simulink model "stm32f0_can_slave_demo"  (Simulink 7.3)
settings: Solver=ode3  SolverMode=SingleTasking  StartTime=0.0  StopTime=10.0  RelTol=1e-3
PreLoadFcn:
  | waijung.modelPreload; % Required for working with Waijung Blockset. Do not remove.
undefined symbols (not defined in the file): current, LQFP48, STM32F072CB, voltage
libraries: stm32f0_can_lib x3, simulink x2, stm32f0_adc_lib x1, stm32f0_device_config_lib x1
CloseFcn:
  | waijung.modelClose; % Required for working with Waijung Blockset. Do not remove.
settings Model: Creator=Krisada  LastModifiedBy=Krisada
settings OptimizationCC: OptimizeModelRefInitCode=on  LifeSpan=1
settings HardwareCC: ProdEndianess=LittleEndian  ProdHWDeviceType=ARM Compatible->Cortex - M0  TargetEndianess=LittleEndian  TargetHWDeviceType=ARM Compatible->Cortex - M0
settings RTWCC: SystemTargetFile=stm32f0.tlc  GenerateMakefile=off  TemplateMakefile=ert_default_tmf  Description=STM32F0 Target  ProcessScript=stm32f0_make_rtw_hook
settings CodeAppCC: IgnoreCustomStorageClasses=off
settings STFCustomTargetCC: ModelReferenceCompliant=off  CombineOutputUpdateFcns=on  ERTCustomFileBanners=on  SupportContinuousTime=off  SupportNonInlinedSFcns=off  SystemTargetFile=stm32f0.tlc
settings ERTTargetCC: MultiwordLength=2048  ModelReferenceCompliant=off  ParMdlRefBuildCompliant=off  CompOptLevelCompliant=off  ERTFirstTimeCompliant=off  ModelStepFunctionPrototypeControlCompliant=off  CPPClassGenCompliant=off  InlinedParameterPlacement=NonHierarchical  ERTSrcFileBannerTemplate=stm32f0_code_template.cgt  ERTHdrFileBannerTemplate=stm32f0_code_template.cgt  ERTDataSrcFileTemplate=stm32f0_code_template.cgt  ERTDataHdrFileTemplate=stm32f0_code_template.cgt  ERTCustomFileTemplate=stm32f0_file_process.tlc

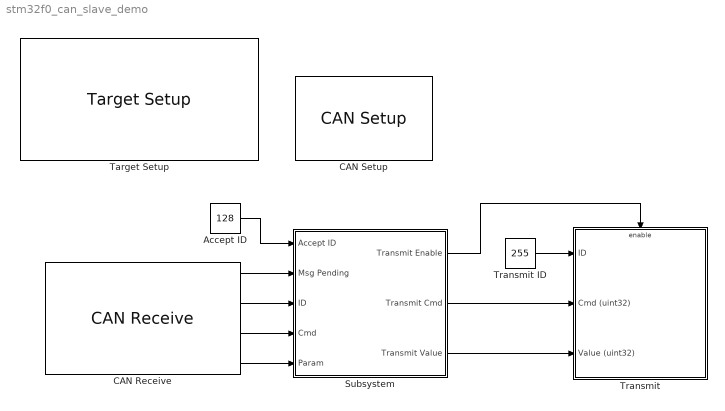
== system stm32f0_can_slave_demo ==
  Accept ID : Constant  Value=128  OutDataTypeMode=uint32  OutDataType=fixdt(1, 16)  OutScaling=2^0  OutDataTypeStr=uint32
  CAN Receive : stm32f0_can_lib/CAN Receive  conf=Rx  canmodule=1  idtype=Standard  filtertype=Mask  id=0  idmask=0  enableisr=off  usedlc=off  datatype=single  data0type=uint32  data1type=uint32  data2type=Not used  data3type=Not used  data4type=Not used  data5type=Not used  data6type=Not used  data7type=Not used  buffersize=8  sampletime=inf  sampletimestr=0.01  blockid=CANReceive  inputarray=[]  inputlabelarray={}  outputarray=[ 5, 7, 7, 7]  outputlabelarray={ 'Msg Pending','ID', 'D0 (uint32)', 'D1 (uint32)' }  compat=0  confstr="[\"Standard\",\"Mask\",\"0\",\"0\",\"off\",\"uint32\",\"uint32\",\"Not used\",\"Not used\",\"Not used\",\"Not used\",\"Not used\",\"Not used\",\"8\",\"0\",\"0\",\"0\",\"4\"]"
  CAN Setup : stm32f0_can_lib/CAN Setup  conf=Setup  canmodule=1  advance=off  bitrate_select=250000  sjw=1tq  bs1=15tq  bs2=8tq  timingconf=Prescaler  brp=8  bitrate=250000  tq=1.6667e-007  autoretransmission=Enable  remaptxpin=B9  remaprxpin=B8  sampletime=-1  sampletimestr=0.01  blockid=CANSetup  inputarray=[]  inputlabelarray={}  outputarray=[]  outputlabelarray={}  compat=0  confstr="[\"250000\",\"8\",\"B\",\"9\",\"B\",\"8\",\"1tq\",\"15tq\",\"8tq\",\"DISABLE\"]"  presc=8  txportstr=B  txpinstr=9  rxportstr=B  rxpinstr=8  lastmodule=1
  Subsystem : Subsystem
  Target Setup : stm32f0_device_config_lib/Target Setup  Priority=100  compiler=GNU ARM  previous_compiler=GNU ARM  mcu=STM32F072CB (LQFP48)  mcustr=STM32F072CB  stdlib=STM32F072  clockconfig=STM32F072B-DISCO Default (HSIOSC-8MHz/HCLK-48MHz)  system_stm32f0xx_c_path=F:\trunk\targets\stm32f0_target\stm32f0\utils\STM32F0xx_AN4055\stm32f0_default\hsi8mhz_pll_hclk48mhz  showmemoryconfiguration=off  stacksize=0x400  heapsize=0x200  enableautocompiledownload=on  fullchiperase=off  programmerinterface=aMG USB Connect  editctrlstr=off  compilercontrolstr=$(patsubst %, -I%, .) -mcpu=cortex-m0 -mthumb -mabi=aapcs -Wall -O3 -mfloat-abi=soft -ffunction-sections -fdata-sections -fno-strict-aliasing -fno-builtin --short-enums  assemblercontrolstr=$(patsubst %, -I%, .) -mcpu=cortex-m0 -mtune=cortex-m0 -mthumb -Wall -O3 -Wa,-amhls=$(<:.s=.lst) -D__STACK_SIZE=$(STACK_SIZE) -D__HEAP_SIZE=$(HEAP_SIZE)  linkercontrolstr="-T$(LD_SCRIPT) -Wl,-Map=$(MAP),--cref,--no-warn-mismatch -mcpu=cortex-m0 -mthumb  -Wall -O3 -mabi=aapcs -lc -specs=nosys.specs"  runafterdownload=on  execprofile=None  profileruart=3  profilerbaud=500000  profilertxpin=Not used  profilerinitstr=0.01,48000000,480000,500000,0  manualsetsampletime=on  sampletime=0.01  blockid=TargetSetup  systickreloadvalue=480000  hseval=8000000  lastprofileruart=3  hclk=48000000  flashorigin=0x8000000  flashlength=128k  ramorigin=0x20000000  ramlength=16k  useextram=off
  Transmit : Subsystem
  Transmit ID : Constant  Value=255  OutDataTypeMode=uint32  OutDataType=fixdt(1, 16)  OutScaling=2^0  OutDataTypeStr=uint32
  wires:
  CAN Receive/1 -> Subsystem/2(Msg Pending)
  CAN Receive/2 -> Subsystem/3(ID)
  CAN Receive/3 -> Subsystem/4(Cmd)
  CAN Receive/4 -> Subsystem/5(Param)
  Accept ID/1 -> Subsystem/1(Accept ID)
  Subsystem/3(Transmit Value) -> Transmit/3(Value (uint32))
  Subsystem/2(Transmit Cmd) -> Transmit/2(Cmd (uint32))
  Subsystem/1(Transmit Enable) -> Transmit/Enable
  Transmit ID/1 -> Transmit/1(ID)

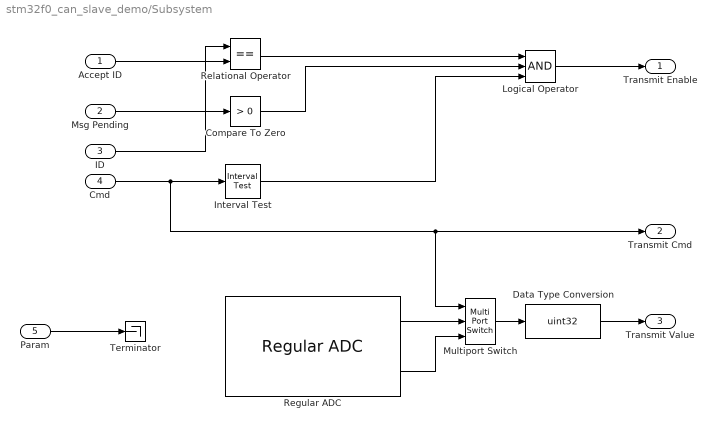
== system stm32f0_can_slave_demo/Subsystem ==
  Accept ID : Inport  OutDataType=fixdt(1, 16)  OutScaling=2^0
  Msg Pending : Inport  Port=2  OutDataType=fixdt(1, 16)  OutScaling=2^0
  ID : Inport  Port=3  OutDataType=fixdt(1, 16)  OutScaling=2^0
  Cmd : Inport  Port=4  OutDataType=fixdt(1, 16)  OutScaling=2^0
  Param : Inport  Port=5  OutDataType=fixdt(1, 16)  OutScaling=2^0
  Compare To Zero : simulink/Logic and Bit Operations/Compare To Zero  SystemSampleTime=-1  relop=>  LogicOutDataTypeMode=uint8  ZeroCross=off
  Data Type Conversion : DataTypeConversion  OutDataTypeMode=uint32  OutDataType=fixdt(1, 16)  OutScaling=2^0  OutDataTypeStr=uint32
  Interval Test : simulink/Logic and Bit Operations/Interval Test  SystemSampleTime=-1  IntervalClosedRight=on  uplimit=1  IntervalClosedLeft=on  lowlimit=0  LogicOutDataTypeMode=uint8
  Logical Operator : Logic  Inputs=3  AllPortsSameDT=off  OutDataTypeMode=boolean  LogicDataType=fixdt(0, 8)  OutDataTypeStr=boolean
  Multiport Switch : MultiPortSwitch  Inputs=2  zeroidx=on  OutDataType=fixdt(1, 16)  OutScaling=2^0
  Regular ADC : stm32f0_adc_lib/Regular ADC  conf=adc  module=1  samplingtime=28.5 Cycles  outputdatatype=Single  adc_ch0=off  adc_ch1=off  adc_ch2=off  adc_ch3=off  adc_ch4=off  adc_ch5=off  adc_ch6=on  adc_ch7=on  adc_ch8=off  adc_ch9=off  adc_ch10=off  adc_ch11=off  adc_ch12=off  adc_ch13=off  adc_ch14=off  adc_ch15=off  adc_ch16=off  adc_ch17=off  adc_ch18=off  sampletime=inf  enablecustomportlabel=off  coutputportlabel=voltage,current  portpinstr=0  blockid=SubsystemRegularADC  inputporttype=[]  inputportwidth=[]  inputportlabel={}  outputporttype=[1 1]  outputportwidth=[]  outputportlabel={'ADC_IN6' 'ADC_IN7'}  compat=0  optionstring="[\"1\",\"ADC_SampleTime_28_5Cycles\",\"dummy\",\"dummy\",\"dummy\",\"0\",\"A\",\"0\",\"0\",\"A\",\"1\",\"0\",\"A\",\"2\",\"0\",\"A\",\"3\",\"0\",\"A\",\"4\",\"0\",\"A\",\"5\",\"1\",\"A\",\"6\",\"1\",\"A\",\"7\",\"0\",\"B\",\"0\",\"0\",\"B\",\"1\",\"0\",\"C\",\"0\",\"0\",\"C\",\"1\",\"0\",\"C\",\"2\",\"0\",\"C\",\"3\",\"0\",\"C\",\"4\",\"0\",\"C\",\"5\",\"0\",\"A\",\"0\",\"0\",\"A\",\"0\",\"0\",\"A\",\"0\",\"2\",\"1\",\"1\",\"1\",\"0\",\"0\",\"0\",\"float\"]"
  Relational Operator : RelationalOperator  Operator===  LogicOutDataTypeMode=boolean  LogicDataType=fixdt(0, 8)  OutDataTypeStr=boolean
  Terminator : Terminator
  Transmit Enable : Outport  OutDataType=fixdt(1, 16)  OutScaling=2^0
  Transmit Cmd : Outport  Port=2  OutDataType=fixdt(1, 16)  OutScaling=2^0
  Transmit Value : Outport  Port=3  OutDataType=fixdt(1, 16)  OutScaling=2^0
  wires:
  Msg Pending/1 -> Compare To Zero/1
  Accept ID/1 -> Relational Operator/2
  ID/1 -> Relational Operator/1
  Cmd/1 -> Interval Test/1, Transmit Cmd/1, Multiport Switch/1
  Relational Operator/1 -> Logical Operator/1
  Compare To Zero/1 -> Logical Operator/2
  Interval Test/1 -> Logical Operator/3
  Logical Operator/1 -> Transmit Enable/1
  Param/1 -> Terminator/1
  Regular ADC/1 -> Multiport Switch/2
  Regular ADC/2 -> Multiport Switch/3
  Multiport Switch/1 -> Data Type Conversion/1
  Data Type Conversion/1 -> Transmit Value/1

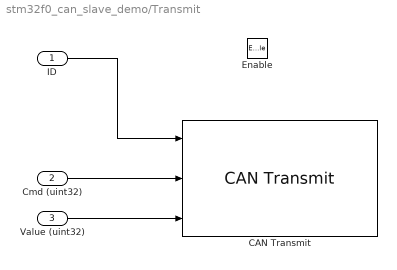
== system stm32f0_can_slave_demo/Transmit ==
  ID : Inport
  Cmd (uint32) : Inport  Port=2
  Value (uint32) : Inport  Port=3
  Enable : EnablePort
  CAN Transmit : stm32f0_can_lib/CAN Transmit  conf=Tx  canmodule=1  transfer=Blocking  timeout=0.1  idtype=Standard  specificid=off  id=0  specificdlc=on  dlc=8  enablestatus=off  datatype=single  data0type=uint32  data1type=uint32  data2type=Not used  data3type=Not used  data4type=Not used  data5type=Not used  data6type=Not used  data7type=Not used  inputarray=[ -1, 7, 7]  inputlabelarray={ 'ID', 'D0 (uint32)', 'D1 (uint32)' }  outputarray=[]  outputlabelarray={}  sampletime=-1  sampletimestr=0.01  blockid=TransmitCANTransmit  compat=0  confstr="[\"Blocking\",\"0.1\",\"Standard\",\"off\",\"0\",\"on\",\"8\",\"off\",\"uint32\",\"uint32\",\"Not used\",\"Not used\",\"Not used\",\"Not used\",\"Not used\",\"Not used\"]"
  wires:
  ID/1 -> CAN Transmit/1
  Cmd (uint32)/1 -> CAN Transmit/2
  Value (uint32)/1 -> CAN Transmit/3
